simulink model "example_1_slx"  (R2021b)
settings: Solver=VariableStepAuto  StartTime=0.0  StopTime=10.0  RelTol=1e-3
undefined symbols (not defined in the file or in its folder): a
settings Model: Creator=yingguang wang  LastModifiedBy=yingguang wang

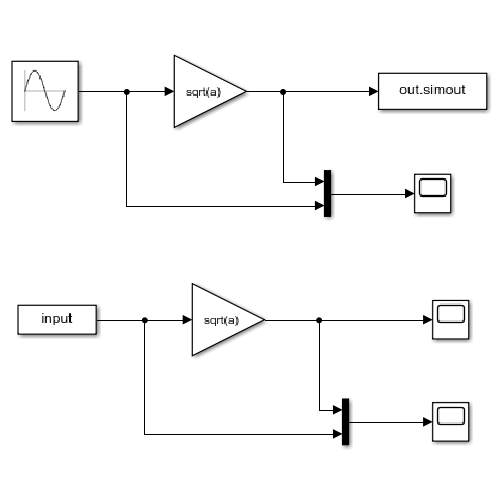
[thumbnail: Simulink's stored preview of the top-level diagram]
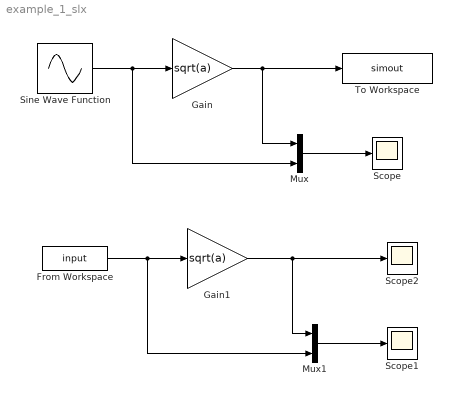
== system example_1_slx ==
  From Workspace : FromWorkspace  VariableName=input
  Gain : Gain  Gain=sqrt(a)
  Gain1 : Gain  Gain=sqrt(a)
  Mux : Mux  Inputs=2
  Mux1 : Mux  Inputs=2
  Scope : Scope
  Scope1 : Scope
  Scope2 : Scope
  Sine Wave Function : Sin  SampleTime=0
  To Workspace : ToWorkspace  VariableName=simout  SaveFormat=Timeseries  SampleTime=-1
  wires:
  Gain/1 -> Mux/1, To Workspace/1
  Mux/1 -> Scope/1
  Sine Wave Function/1 -> Gain/1, Mux/2
  From Workspace/1 -> Gain1/1, Mux1/2
  Mux1/1 -> Scope1/1
  Gain1/1 -> Scope2/1, Mux1/1
